simulink model "excercise1_3bd1"  (R2023b)
settings: Solver=VariableStepAuto  StartTime=0.0  StopTime=3  RelTol=1e-3
undefined symbols (not defined in the file): d, k, m
settings Model: Creator=elliot  LastModifiedBy=elliot

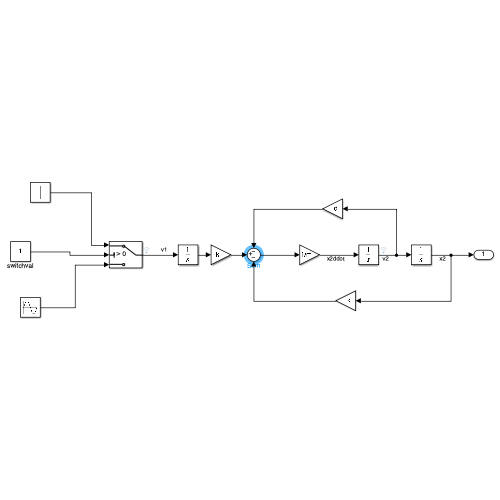
[thumbnail: Simulink's stored preview of the top-level diagram]
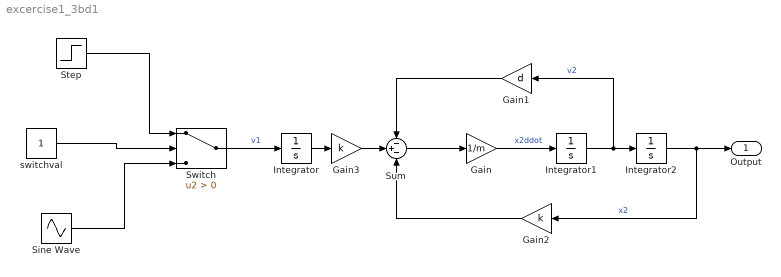
== system excercise1_3bd1 ==
  Gain : Gain  Gain=1/m
  Gain1 : Gain  Gain=d
  Gain2 : Gain  Gain=k
  Gain3 : Gain  Gain=k
  Integrator : Integrator
  Integrator1 : Integrator
  Integrator2 : Integrator
  Sine Wave : Sin  Frequency=20  SampleTime=0
  Step : Step  SampleTime=0
  Sum : Sum  Inputs=-+-
  Switch : Switch  Criteria=u2 > Threshold  SaturateOnIntegerOverflow=off  InputSameDT=off
  switchval : Constant
  Output : Outport
  wires:
  switchval/1 -> Switch/2
  Step/1 -> Switch/1
  Switch/1 -> Integrator/1  "v1"
  Sine Wave/1 -> Switch/3
  Sum/1 -> Gain/1
  Gain/1 -> Integrator1/1  "x2ddot"
  Integrator1/1 -> Gain1/1, Integrator2/1  "v2"
  Integrator2/1 -> Gain2/1, Output/1  "x2"
  Gain1/1 -> Sum/1
  Gain2/1 -> Sum/3
  Integrator/1 -> Gain3/1
  Gain3/1 -> Sum/2
